simulink model "sl_vloop_test"  (R2022a)
settings: Solver=ode15s  StartTime=0.0  StopTime=1.0  RelTol=1e-3  EnableMultiTasking=on
InitFcn:
  | G = 107.815;
libraries: roblocks x1, simulink x1
Description:
  | Test harness for joint velocity control loop for
  | PUMA 560 shoulder joint with link inertia
  | 
  | Robotics, Vision and Control - 3rd Edition; Section 9.1.6
settings Model: DisableUpgradeWarningsForVersion=R2014b  Creator=pic  LastModifiedBy=rpill
settings SolverCC: AlgebraicLoopSolver=TrustRegion  MaxZcPerStep=1
settings DataIOCC: LimitDataPoints=on  SaveFormat=Array  SignalLoggingSaveFormat=ModelDataLogs  TimeSaveName=t  OutputSaveName=y
settings OptimizationCC: ExpressionDepthLimit=2147483647  LifeSpan=inf
settings DebuggingCC: UnderspecifiedInitializationDetection=Classic  MergeDetectMultiDrivingBlocksExec=none  SolverPrmCheckMsg=warning  MultiTaskRateTransMsg=warning  FcnCallInpInsideContextMsg=warning  UnconnectedInputMsg=warning  UnconnectedOutputMsg=warning  UnconnectedLineMsg=warning  AllowSymbolicDim=off  StateNameClashWarn=warning  SFUnexpectedBacktrackingDiag=warning  SFNoUnconditionalDefaultTransitionDiag=warning  SFExecutionAtInitializationDiag=none  SFMachineParentedDataDiag=warning  ArithmeticOperatorsInVariantConditions=warning
settings HardwareCC: ProdBitPerPointer=32  ProdBitPerSizeT=32  ProdBitPerPtrDiffT=32  ProdLargestAtomicFloat=None  ProdIntDivRoundTo=Undefined  ProdEndianess=Unspecified  ProdWordSize=32  ProdHWDeviceType=32-bit Generic
settings ModelReferenceCC: PropagateSignalLabelsOutOfModel=off
settings SFSimCC: SimUseLocalCustomCode=off  CustomCodeUndefinedFunction=UseInterfaceOnly
settings SFSimCC: SimCustomInitializer=|
  | if ~exist(tau_d)
  |    tau_d = 0
  | end
settings RTWCC: RTWUseLocalCustomCode=off
settings CodeAppCC: StateflowObjectComments=on
settings GRTTargetCC: TargetLangStandard=C89/C90 (ANSI)  CombineOutputUpdateFcns=off  GRTInterface=on
settings ConfigComp: CovMetricSettings=dw  CovSaveCumulativeToWorkspaceVar=on  CovSaveSingleToWorkspaceVar=on  CovExternalEMLEnable=off  CovSFcnEnable=off

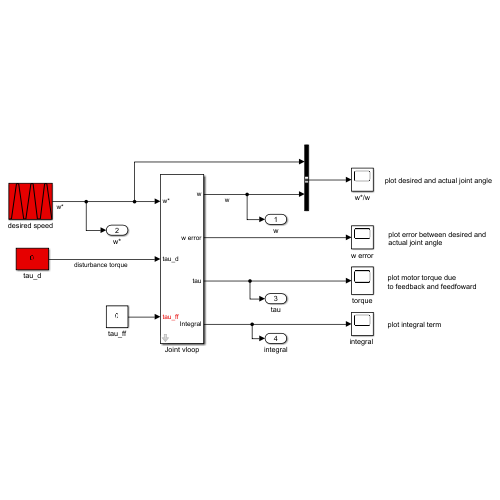
[thumbnail: Simulink's stored preview of the top-level diagram]
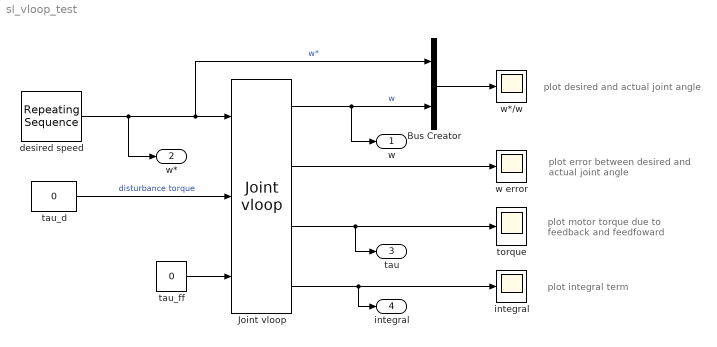
== system sl_vloop_test ==
  note: plot integral term
  note: plot motor torque due
      | to feedback and feedfoward
  note: plot error between desired and
      | actual joint angle
  note: plot desired and actual joint angle
  Bus Creator : BusCreator  Inputs=2
  Joint vloop : roblocks/Joint vloop  J=580e-6  B=817e-6  Km=0.228  tau_max=0.9  Kv=0.6  Ki=0  T=0.001
  desired speed : simulink/Sources/Repeating Sequence  rep_seq_t=[0 1 3 4 6]/10  rep_seq_y=[0 0 50 50 0]
  "integral " : Scope
  tau_d : Constant  Value=0
  tau_ff : Constant  Value=0
  torque : Scope
  w error : Scope
  w*/w : Scope
  w : Outport
  w* : Outport  Port=2
  tau : Outport  Port=3
  integral : Outport  Port=4
  wires:
  desired speed/1 -> w*/1, Joint vloop/1, Bus Creator/1  "w*"
  Bus Creator/1 -> w*/w/1
  Joint vloop/1 -> Bus Creator/2, w/1  "w"
  Joint vloop/2 -> w error/1
  Joint vloop/3 -> tau/1, torque/1
  Joint vloop/4 -> integral/1, "integral "/1
  tau_d/1 -> Joint vloop/2  "disturbance torque"
  tau_ff/1 -> Joint vloop/3
